simulink model "find6DOFSnellMin9_th"  (R2018b)
settings: Solver=ode8  StartTime=0.0  StopTime=len  FixedStep=1  RelTol=1e-3  EnableMultiTasking=on
undefined symbols (not defined in the file or in its folder): cam1Dot1, cam1Dot2, cam1Dot3, cam2Dot1, cam2Dot2, cam2Dot3, cam3Dot1, cam3Dot2, cam3Dot3
libraries: find6DOFSnellMin9_cl x1
settings Model: Creator=MAE-NCSUCORE  LastModifiedBy=MAE-NCSUCORE
settings SolverCC: ConcurrentTasks=on  AutoInsertRateTranBlk=on
settings DataIOCC: SaveFormat=StructureWithTime
settings OptimizationCC: BlockReduction=off  OptimizeBlockIOStorage=off  BufferReuse=off  GlobalBufferReuse=off  ExpressionFolding=off  LocalBlockOutputs=off  OptimizeDataStoreBuffers=off  BusAssignmentInplaceUpdate=off
settings DebuggingCC: UnitsInconsistencyMsg=none
settings HardwareCC: ProdBitPerPointer=32  ProdBitPerSizeT=32  ProdBitPerPtrDiffT=32  ProdLargestAtomicFloat=None  ProdWordSize=32  ProdLongLongMode=on  ProdHWDeviceType=Generic->32-bit x86 compatible
settings RTWCC: Description=Generic Real-Time Target  RTWCompilerOptimization=on
settings GRTTargetCC: TargetLangStandard=C89/C90 (ANSI)

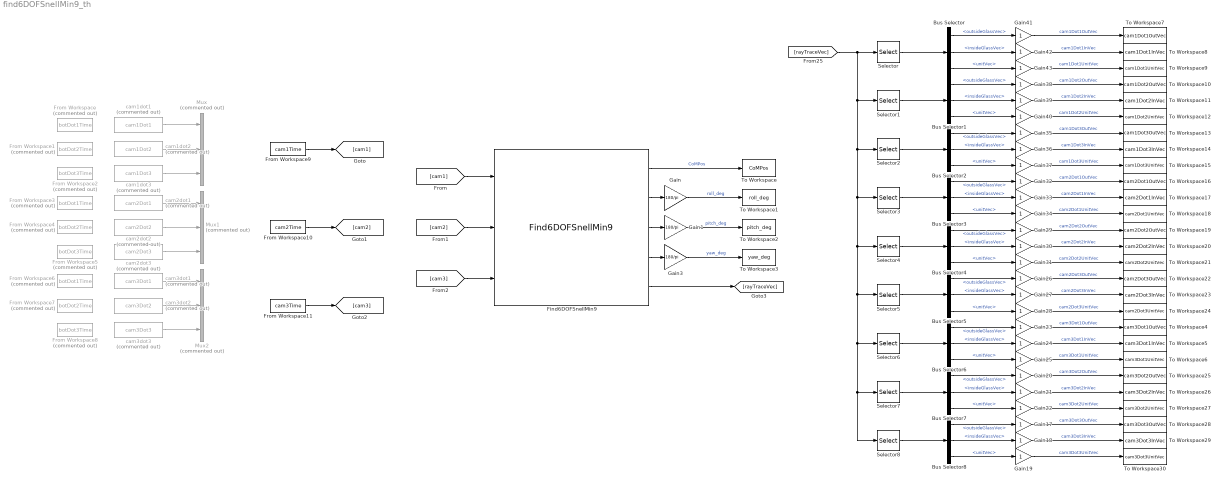
== system find6DOFSnellMin9_th ==
  Bus Selector{,1..8} (9 alike) : BusSelector  OutputSignals=outsideGlassVec,insideGlassVec,unitVec
  Find6DOFSnellMin9 : find6DOFSnellMin9_cl/Find6DOFSnellMin9  imageDims_px=params.sideImageSize_px.Value  initialCoMPositionVec_cm=params.initCoMPosVec_cm.Value  initialEulerAngles_deg=params.initEulerAng_deg.Value  indxOfRefVec=params.indexOfRefractionA.Value  glassThickness_cm=params.glassThickness_cm.Value  snells=snells  glassPlane=1  cameraFOVAngles_deg=params.cameraFOV_deg.Value  sideEulerAngles_deg=params.sideCamEulAng_deg.Value  sideCamPositionVec_cm=params.sideCamPosVec_cm.Value  sideCamDistToGlass_cm=params.sideDistancetoGlass_cm.Value  botEulerAngles_deg=params.botCamEulAng_deg.Value  botCamPositionVec_cm=params.botCamPosVec_cm.Value  botCamDistToGlass_cm=params.botDistancetoGlass_cm.Value  slantEulerAngles_deg=params.slntCamEulAng_deg.Value  slantCamPositionVec_cm=params.slntCamPosVec_cm.Value  slantCamDistToGlass_cm=params.slntDistancetoGlass_cm.Value  sideSeparation_cm=params.sideDotSepDist_cm.Value  sidePositionVecBF_cm=params.sideDotPosVec_cm.Value  bottomASeparation_cm=params.botADotSepDist_cm.Value  botAPositionVecBF_cm=params.botADotPosVec_cm.Value  bottomBSeparation_cm=params.botBDotSepDist_cm.Value  botBPositionVecBF_cm=params.botBDotPosVec_cm.Value
  From Workspace : FromWorkspace  Commented=on  VariableName=botDot1Time  SampleTime=0
  From Workspace1 : FromWorkspace  Commented=on  VariableName=botDot2Time  SampleTime=0
  From Workspace10 : FromWorkspace  VariableName=cam2Time  SampleTime=0
  From Workspace11 : FromWorkspace  VariableName=cam3Time  SampleTime=0
  From Workspace2 : FromWorkspace  Commented=on  VariableName=botDot3Time  SampleTime=0
  From Workspace3 : FromWorkspace  Commented=on  VariableName=botDot1Time  SampleTime=0
  From Workspace4 : FromWorkspace  Commented=on  VariableName=botDot2Time  SampleTime=0
  From Workspace5 : FromWorkspace  Commented=on  VariableName=botDot3Time  SampleTime=0
  From Workspace6 : FromWorkspace  Commented=on  VariableName=botDot1Time  SampleTime=0
  From Workspace7 : FromWorkspace  Commented=on  VariableName=botDot2Time  SampleTime=0
  From Workspace8 : FromWorkspace  Commented=on  VariableName=botDot3Time  SampleTime=0
  From Workspace9 : FromWorkspace  VariableName=cam1Time  SampleTime=0
  Gain : Gain  Gain=180/pi
  Gain1 : Gain  Gain=180/pi
  Gain{17..43} (27 alike) : Gain
  Gain3 : Gain  Gain=180/pi
  Mux : Mux  Commented=on  Inputs=3
  Mux1 : Mux  Commented=on  Inputs=3
  Mux2 : Mux  Commented=on  Inputs=3
  Selector : Selector  InputPortWidth=9  IndexOptions=Index vector (dialog)  Indices=[1]  OutputSizes=1
  Selector1 : Selector  InputPortWidth=9  IndexOptions=Index vector (dialog)  Indices=[2]  OutputSizes=1
  Selector2 : Selector  InputPortWidth=9  IndexOptions=Index vector (dialog)  Indices=[3]  OutputSizes=1
  Selector3 : Selector  InputPortWidth=9  IndexOptions=Index vector (dialog)  Indices=[4]  OutputSizes=1
  Selector4 : Selector  InputPortWidth=9  IndexOptions=Index vector (dialog)  Indices=[5]  OutputSizes=1
  Selector5 : Selector  InputPortWidth=9  IndexOptions=Index vector (dialog)  Indices=[6]  OutputSizes=1
  Selector6 : Selector  InputPortWidth=9  IndexOptions=Index vector (dialog)  Indices=[7]  OutputSizes=1
  Selector7 : Selector  InputPortWidth=9  IndexOptions=Index vector (dialog)  Indices=[8]  OutputSizes=1
  Selector8 : Selector  InputPortWidth=9  IndexOptions=Index vector (dialog)  Indices=[9]  OutputSizes=1
  To Workspace : ToWorkspace  VariableName=CoMPos  SaveFormat=Timeseries  SampleTime=-1
  To Workspace1 : ToWorkspace  VariableName=roll_deg  SaveFormat=Timeseries  SampleTime=-1
  To Workspace10 : ToWorkspace  VariableName=cam1Dot2OutVec  SaveFormat=Timeseries  SampleTime=-1
  To Workspace11 : ToWorkspace  VariableName=cam1Dot2InVec  SaveFormat=Timeseries  SampleTime=-1
  To Workspace12 : ToWorkspace  VariableName=cam1Dot2UnitVec  SaveFormat=Timeseries  SampleTime=-1
  To Workspace13 : ToWorkspace  VariableName=cam1Dot3OutVec  SaveFormat=Timeseries  SampleTime=-1
  To Workspace14 : ToWorkspace  VariableName=cam1Dot3InVec  SaveFormat=Timeseries  SampleTime=-1
  To Workspace15 : ToWorkspace  VariableName=cam1Dot3UnitVec  SaveFormat=Timeseries  SampleTime=-1
  To Workspace16 : ToWorkspace  VariableName=cam2Dot1OutVec  SaveFormat=Timeseries  SampleTime=-1
  To Workspace17 : ToWorkspace  VariableName=cam2Dot1InVec  SaveFormat=Timeseries  SampleTime=-1
  To Workspace18 : ToWorkspace  VariableName=cam2Dot1UnitVec  SaveFormat=Timeseries  SampleTime=-1
  To Workspace19 : ToWorkspace  VariableName=cam2Dot2OutVec  SaveFormat=Timeseries  SampleTime=-1
  To Workspace2 : ToWorkspace  VariableName=pitch_deg  SaveFormat=Timeseries  SampleTime=-1
  To Workspace20 : ToWorkspace  VariableName=cam2Dot2InVec  SaveFormat=Timeseries  SampleTime=-1
  To Workspace21 : ToWorkspace  VariableName=cam2Dot2UnitVec  SaveFormat=Timeseries  SampleTime=-1
  To Workspace22 : ToWorkspace  VariableName=cam2Dot3OutVec  SaveFormat=Timeseries  SampleTime=-1
  To Workspace23 : ToWorkspace  VariableName=cam2Dot3InVec  SaveFormat=Timeseries  SampleTime=-1
  To Workspace24 : ToWorkspace  VariableName=cam2Dot3UnitVec  SaveFormat=Timeseries  SampleTime=-1
  To Workspace25 : ToWorkspace  VariableName=cam3Dot2OutVec  SaveFormat=Timeseries  SampleTime=-1
  To Workspace26 : ToWorkspace  VariableName=cam3Dot2InVec  SaveFormat=Timeseries  SampleTime=-1
  To Workspace27 : ToWorkspace  VariableName=cam3Dot2UnitVec  SaveFormat=Timeseries  SampleTime=-1
  To Workspace28 : ToWorkspace  VariableName=cam3Dot3OutVec  SaveFormat=Timeseries  SampleTime=-1
  To Workspace29 : ToWorkspace  VariableName=cam3Dot3InVec  SaveFormat=Timeseries  SampleTime=-1
  To Workspace3 : ToWorkspace  VariableName=yaw_deg  SaveFormat=Timeseries  SampleTime=-1
  To Workspace30 : ToWorkspace  VariableName=cam3Dot3UnitVec  SaveFormat=Timeseries  SampleTime=-1
  To Workspace4 : ToWorkspace  VariableName=cam3Dot1OutVec  SaveFormat=Timeseries  SampleTime=-1
  To Workspace5 : ToWorkspace  VariableName=cam3Dot1InVec  SaveFormat=Timeseries  SampleTime=-1
  To Workspace6 : ToWorkspace  VariableName=cam3Dot1UnitVec  SaveFormat=Timeseries  SampleTime=-1
  To Workspace7 : ToWorkspace  VariableName=cam1Dot1OutVec  SaveFormat=Timeseries  SampleTime=-1
  To Workspace8 : ToWorkspace  VariableName=cam1Dot1InVec  SaveFormat=Timeseries  SampleTime=-1
  To Workspace9 : ToWorkspace  VariableName=cam1Dot1UnitVec  SaveFormat=Timeseries  SampleTime=-1
  cam1dot1 : Constant  Commented=on  Value=cam1Dot1
  cam1dot2 : Constant  Commented=on  Value=cam1Dot2
  cam1dot3 : Constant  Commented=on  Value=cam1Dot3
  cam2dot1 : Constant  Commented=on  Value=cam2Dot1
  cam2dot2 : Constant  Commented=on  Value=cam2Dot2
  cam2dot3 : Constant  Commented=on  Value=cam2Dot3
  cam3dot1 : Constant  Commented=on  Value=cam3Dot1
  cam3dot2 : Constant  Commented=on  Value=cam3Dot2
  cam3dot3 : Constant  Commented=on  Value=cam3Dot3
  wires:
  [cam1] -> Find6DOFSnellMin9/1
  [cam2] -> Find6DOFSnellMin9/2
  [cam3] -> Find6DOFSnellMin9/3
  Find6DOFSnellMin9/1 -> To Workspace/1  "CoMPos"
  Find6DOFSnellMin9/2 -> Gain/1
  Gain/1 -> To Workspace1/1  "roll_deg"
  Find6DOFSnellMin9/3 -> Gain1/1
  Gain1/1 -> To Workspace2/1  "pitch_deg"
  Find6DOFSnellMin9/4 -> Gain3/1
  Gain3/1 -> To Workspace3/1  "yaw_deg"
  cam1dot1/1 -> Mux/1
  cam1dot2/1 -> Mux/2
  cam1dot3/1 -> Mux/3
  cam2dot1/1 -> Mux1/1
  cam2dot2/1 -> Mux1/2
  cam2dot3/1 -> Mux1/3
  cam3dot1/1 -> Mux2/1
  cam3dot2/1 -> Mux2/2
  cam3dot3/1 -> Mux2/3
  From Workspace11/1 -> [cam3]
  From Workspace10/1 -> [cam2]
  From Workspace9/1 -> [cam1]
  Gain19/1 -> To Workspace30/1  "cam3Dot3UnitVec"
  Gain29/1 -> To Workspace19/1  "cam2Dot2OutVec"
  Gain23/1 -> To Workspace4/1  "cam3Dot1OutVec"
  Gain31/1 -> To Workspace21/1  "cam2Dot2UnitVec"
  Gain33/1 -> To Workspace17/1  "cam2Dot1InVec"
  Gain20/1 -> To Workspace25/1  "cam3Dot2OutVec"
  Selector6/1 -> Bus Selector6/1
  Bus Selector4/2 -> Gain30/1  "<insideGlassVec>"
  Bus Selector5/2 -> Gain27/1  "<insideGlassVec>"
  Bus Selector/1 -> Gain41/1  "<outsideGlassVec>"
  Bus Selector/2 -> Gain42/1  "<insideGlassVec>"
  Gain41/1 -> To Workspace7/1  "cam1Dot1OutVec"
  Bus Selector6/1 -> Gain23/1  "<outsideGlassVec>"
  Gain37/1 -> To Workspace15/1  "cam1Dot3UnitVec"
  Gain18/1 -> To Workspace29/1  "cam3Dot3InVec"
  Bus Selector1/1 -> Gain38/1  "<outsideGlassVec>"
  Gain28/1 -> To Workspace24/1  "cam2Dot3UnitVec"
  Gain27/1 -> To Workspace23/1  "cam2Dot3InVec"
  Bus Selector2/2 -> Gain36/1  "<insideGlassVec>"
  Gain34/1 -> To Workspace18/1  "cam2Dot1UnitVec"
  Bus Selector7/3 -> Gain22/1  "<unitVec>"
  Gain35/1 -> To Workspace13/1  "cam1Dot3OutVec"
  Bus Selector7/1 -> Gain20/1  "<outsideGlassVec>"
  Gain22/1 -> To Workspace27/1  "cam3Dot2UnitVec"
  Gain43/1 -> To Workspace9/1  "cam1Dot1UnitVec"
  Gain24/1 -> To Workspace5/1  "cam3Dot1InVec"
  Gain32/1 -> To Workspace16/1  "cam2Dot1OutVec"
  Gain42/1 -> To Workspace8/1  "cam1Dot1InVec"
  Bus Selector4/1 -> Gain29/1  "<outsideGlassVec>"
  Bus Selector5/3 -> Gain28/1  "<unitVec>"
  Bus Selector2/3 -> Gain37/1  "<unitVec>"
  Gain36/1 -> To Workspace14/1  "cam1Dot3InVec"
  Bus Selector8/2 -> Gain18/1  "<insideGlassVec>"
  Bus Selector1/2 -> Gain39/1  "<insideGlassVec>"
  Selector3/1 -> Bus Selector3/1
  Selector2/1 -> Bus Selector2/1
  Bus Selector3/3 -> Gain34/1  "<unitVec>"
  Bus Selector3/2 -> Gain33/1  "<insideGlassVec>"
  Selector4/1 -> Bus Selector4/1
  Selector/1 -> Bus Selector/1
  Bus Selector3/1 -> Gain32/1  "<outsideGlassVec>"
  Gain38/1 -> To Workspace10/1  "cam1Dot2OutVec"
  Bus Selector4/3 -> Gain31/1  "<unitVec>"
  Gain40/1 -> To Workspace12/1  "cam1Dot2UnitVec"
  Gain17/1 -> To Workspace28/1  "cam3Dot3OutVec"
  Gain25/1 -> To Workspace6/1  "cam3Dot1UnitVec"
  Gain21/1 -> To Workspace26/1  "cam3Dot2InVec"
  Bus Selector6/2 -> Gain24/1  "<insideGlassVec>"
  Bus Selector6/3 -> Gain25/1  "<unitVec>"
  Bus Selector8/3 -> Gain19/1  "<unitVec>"
  Selector7/1 -> Bus Selector7/1
  Selector5/1 -> Bus Selector5/1
  Gain39/1 -> To Workspace11/1  "cam1Dot2InVec"
  Selector8/1 -> Bus Selector8/1
  Bus Selector1/3 -> Gain40/1  "<unitVec>"
  Gain30/1 -> To Workspace20/1  "cam2Dot2InVec"
  Bus Selector/3 -> Gain43/1  "<unitVec>"
  Selector1/1 -> Bus Selector1/1
  Bus Selector5/1 -> Gain26/1  "<outsideGlassVec>"
  Bus Selector8/1 -> Gain17/1  "<outsideGlassVec>"
  Gain26/1 -> To Workspace22/1  "cam2Dot3OutVec"
  Bus Selector2/1 -> Gain35/1  "<outsideGlassVec>"
  Bus Selector7/2 -> Gain21/1  "<insideGlassVec>"
  Find6DOFSnellMin9/5 -> [rayTraceVec]
  [rayTraceVec] -> Selector8/1, Selector7/1, Selector6/1, Selector5/1, Selector4/1, Selector3/1, Selector2/1, Selector1/1, Selector/1
